simulink model "NLE_DataCollection"  (R2024b)
settings: Solver=VariableStepAuto  StartTime=0.0  StopTime=20.0  RelTol=1e-3
values from neighbouring files (symbols this model uses):
  discrete_regulator = tf(Q, P, Ts)    [assignment3.m]
  Ts = 0.75    [assignment3.m]
libraries: simulink x2
settings Model: Creator=lukiq  LastModifiedBy=lukiq
settings DebuggingCC: AlgebraicLoopMsg=none

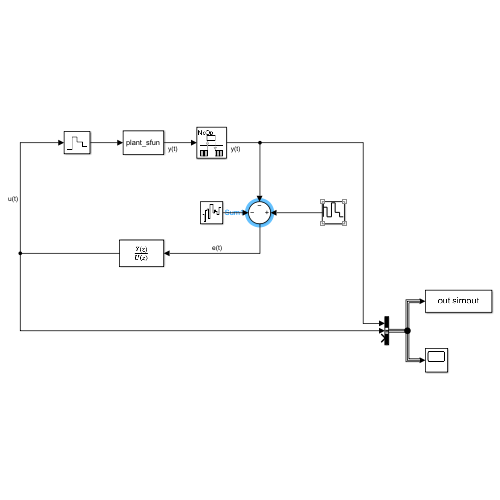
[thumbnail: Simulink's stored preview of the top-level diagram]
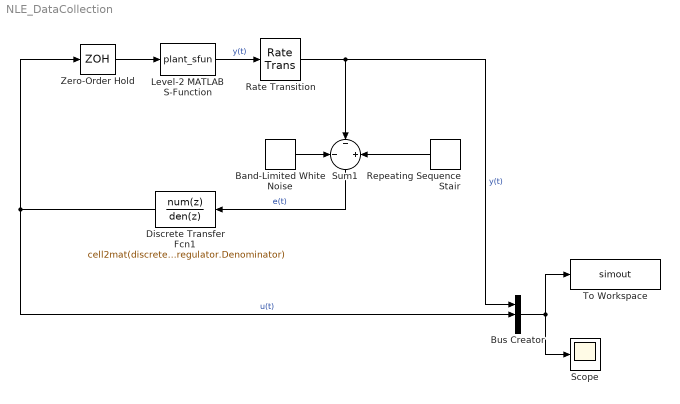
== system NLE_DataCollection ==
  Band-Limited White Noise : simulink/Sources/Band-Limited White Noise  Cov=[0.0001]  Ts=Ts  seed=[23341]
  Bus Creator : BusCreator  Inputs=3
  Discrete Transfer Fcn1 : DiscreteTransferFcn  Numerator=cell2mat(discrete_regulator.Numerator)  Denominator=cell2mat(discrete_regulator.Denominator)
  Level-2 MATLAB S-Function : M-S-Function  FunctionName=plant_sfun  Parameters=odeHandleSimulink, p, u, outIdx
  Rate Transition : RateTransition
  Repeating Sequence Stair : simulink/Sources/Repeating Sequence Stair  OutValues=u_control  tsamp=-1  OutMin=[]  OutMax=[]  OutDataTypeStr=double  OutputDataTypeScalingMode=double  OutDataType=fixdt(0,8)  ConRadixGroup=Best Precision: Vector-wise  OutScaling=2^-12
  Scope : Scope
  Sum1 : Sum  Inputs=-|-|+
  To Workspace : ToWorkspace  VariableName=simout  SaveFormat=Timeseries  SampleTime=-1
  Zero-Order Hold : ZeroOrderHold  SampleTime=-1
  wires:
  Discrete Transfer Fcn1/1 -> Zero-Order Hold/1, Bus Creator/2  "u(t)"
  Repeating Sequence Stair/1 -> Sum1/3
  Sum1/1 -> Discrete Transfer Fcn1/1  "e(t)"
  Rate Transition/1 -> Sum1/2, Bus Creator/1  "y(t)"
  Bus Creator/1 -> Scope/1, To Workspace/1
  Zero-Order Hold/1 -> Level-2 MATLAB S-Function/1
  Level-2 MATLAB S-Function/1 -> Rate Transition/1  "y(t)"
  Band-Limited White Noise/1 -> Sum1/1
